simulink model "task3"  (R2017a)
settings: Solver=VariableStepAuto  StartTime=0.0  StopTime=w_base  MaxStep=1e-4*w_base  RelTol=1e-3
values from neighbouring files (symbols this model uses):
  I_base = 1    [parameters.m]
  K = sqrt(3/2)    [parameters.m]    (also in working.m)
  ki = alpha_c*(R+Ra)    (= 11.8344493889)    [parameters.m]
  ki_speed = alpha_speed*alpha_speed*J    (= 24.390868485)    [parameters.m]
  kp = alpha_c*Lsigma    (= 1.69441359229)    [parameters.m]
  kp_speed = alpha_speed*J    (= 34.9219619187)    [parameters.m]
  LM = 1.301    [parameters.m]
  Lsigma = 0.2426    [parameters.m]
  Ra = alpha_c*Lsigma-R    (= 1.58785359229)    [parameters.m]
  Ra_speed = alpha_speed*J-b    (= 34.4219619187)    [parameters.m]
  Tr = LM/RR    (= 21.1510323525)    [parameters.m]
  V_base = 1    [parameters.m]
settings Model: Creator=Oskar  LastModifiedBy=Callum

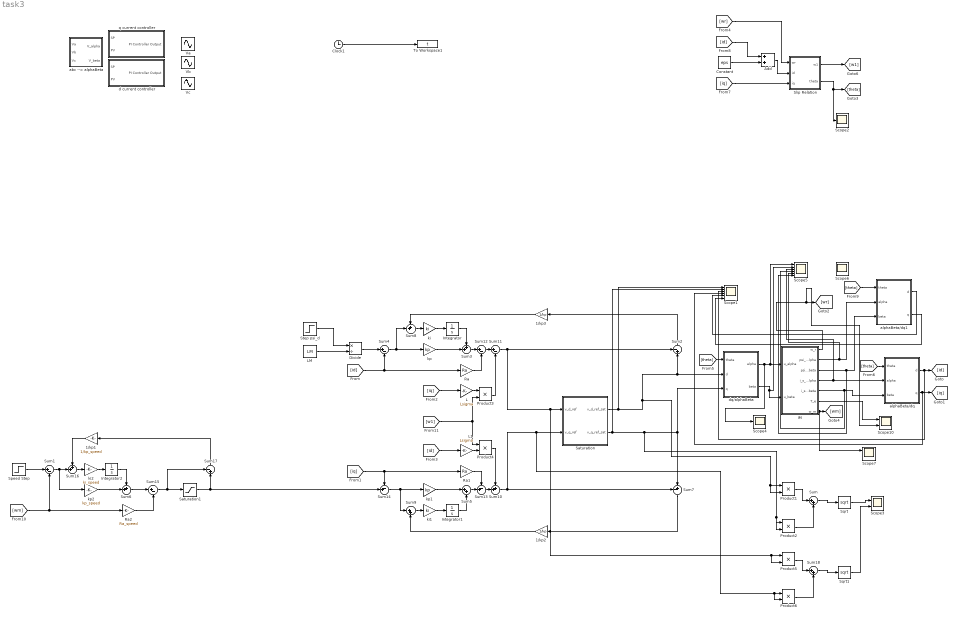
== system task3 ==
  1/kp1 : Gain  Gain=1/kp_speed
  1/kp2 : Gain  Gain=1/kp
  1/kp3 : Gain  Gain=1/kp
  Add : Sum
  Clock1 : Clock
  Constant : Constant  Value=eps
  Divide : Product  Inputs=*/
  IM : Subsystem  mask{RR=0.06151, RS=0.04505, LM=1.301, Ls=0.2426, J=50, p=2, b_w1=0.5, b_w2=0}
      mask prompts: RR "Rr [p.u]"; RS "Rs [p.u]"; LM "Lm [p.u]"; Ls "Ls [p.u]"; J "J [p.u]"
  Integrator : Integrator
  Integrator1 : Integrator
  Integrator2 : Integrator
  L : Gain  Gain=Lsigma
  L1 : Gain  Gain=Lsigma
  LM : Constant  Value=LM
  Product{1..6} (6 alike) : Product
  Ra : Gain  Gain=Ra
  Ra1 : Gain  Gain=Ra
  Ra2 : Gain  Gain=Ra_speed
  Saturation : Subsystem
  Saturation1 : Saturate  UpperLimit=I_base  LowerLimit=-I_base
  Scope1 : Scope  NumInputPorts=6
  Scope10 : Scope  NumInputPorts=2
  Scope2 : Scope
  Scope3 : Scope  NumInputPorts=2
  Scope4 : Scope
  Scope5 : Scope  NumInputPorts=6
  Scope6 : Scope
  Scope7 : Scope  NumInputPorts=2
  Slip Relation : Subsystem
  Speed Step : Step  Time=150  After=0.3  SampleTime=0
  Sqrt : Sqrt  SaturateOnIntegerOverflow=on
  Sqrt1 : Sqrt  SaturateOnIntegerOverflow=on
  Step psi_d : Step  Time=0  Before=1  SampleTime=0
  Sum{,5,9,18} (4 alike) : Sum  Inputs=|++
  Sum{1,4,11..12,15} (5 alike) : Sum  Inputs=|+-
  Sum{3,6,8,10,16} (5 alike) : Sum  Inputs=++|
  Sum{2,7,13..14,17} (5 alike) : Sum  Inputs=-+|
  To Workspace1 : ToWorkspace  VariableName=t
      settings: MaxDataPoints=100000
  Va : Sin  SampleTime=0
  Vb : Sin  Phase=2*pi/3  SampleTime=0
  Vc : Sin  Phase=4*pi/3  SampleTime=0
  abc --> alphaBeta : Subsystem
  alphaBeta/dq : Subsystem
  alphaBeta/dq1 : Subsystem
  d current controller : Subsystem
  dq/alphaBeta : Subsystem
  ki : Gain  Gain=ki
  ki1 : Gain  Gain=ki
  ki2 : Gain  Gain=ki_speed
  kp : Gain  Gain=kp
  kp1 : Gain  Gain=kp
  kp2 : Gain  Gain=kp_speed
  q current controller : Subsystem
  wires:
  Clock1/1 -> To Workspace1/1
  dq/alphaBeta/1(alpha) -> Scope4/1, Scope5/1, IM/1(u_alpha)
  dq/alphaBeta/2(beta) -> Scope5/2, IM/2(u_beta)
  IM/4(i_s_s_alpha) -> Scope5/3, alphaBeta/dq/2(alpha)
  IM/5(i_s_s_beta) -> Scope5/4, alphaBeta/dq/3("beta ")
  alphaBeta/dq/1(d) -> Scope1/3, [id]
  ki/1 -> Integrator/1
  Sum4/1 -> kp/1, Sum8/2
  [id] -> Ra/1, Sum4/2
  Sum14/1 -> kp1/1, Sum9/1
  ki1/1 -> Integrator1/1
  kp1/1 -> Sum5/1
  Integrator1/1 -> Sum5/2
  Sum7/1 -> 1/kp2/1
  Sum2/1 -> 1/kp3/1
  kp/1 -> Sum3/2
  Integrator/1 -> Sum3/1
  Sum8/1 -> ki/1
  1/kp3/1 -> Sum8/1
  Sum9/1 -> ki1/1
  1/kp2/1 -> Sum9/2
  Sum11/1 -> Product5/2, Product5/1, Saturation/1(v_d_ref), Sum2/1
  [iq] -> L/1
  Sum10/1 -> Product6/2, Product6/1, Saturation/2(v_q_ref), Sum7/1
  [id] -> L1/1
  Sum3/1 -> Sum12/1
  Sum12/1 -> Sum11/1
  Ra/1 -> Sum12/2
  Sum5/1 -> Sum13/2
  Sum13/1 -> Sum10/2
  Ra1/1 -> Sum13/1
  [iq] -> Ra1/1, Sum14/1
  [wr] -> Slip Relation/1(wr)
  Slip Relation/2(theta) -> Scope2/1, [theta]
  [theta] -> dq/alphaBeta/1(theta)
  [theta] -> alphaBeta/dq/1(theta)
  [iq] -> Slip Relation/3("iq ")
  L/1 -> Product3/1
  Product3/1 -> Sum11/2
  [w1] -> Product3/2, Product4/1
  L1/1 -> Product4/2
  Product4/1 -> Sum10/1
  Saturation/2(v_q_ref_sat) -> Product2/2, Product2/1, dq/alphaBeta/3("q "), Sum7/2, Scope1/2
  IM/2(psi_r_alpha) -> Scope5/5, alphaBeta/dq1/2(alpha)
  IM/3(psi_r_beta) -> Scope5/6, alphaBeta/dq1/3("beta ")
  [theta] -> alphaBeta/dq1/1(theta)
  Slip Relation/1(w1) -> [w1]
  Add/1 -> Slip Relation/2(id)
  Constant/1 -> Add/2
  [id] -> Add/1
  Speed Step/1 -> Sum1/1
  [wm] -> Sum1/2, Ra2/1
  ki2/1 -> Integrator2/1
  Sum16/1 -> ki2/1
  kp2/1 -> Sum6/2
  Integrator2/1 -> Sum6/1
  Sum1/1 -> kp2/1, Sum16/2
  Sum6/1 -> Sum15/1
  Ra2/1 -> Sum15/2
  1/kp1/1 -> Sum16/1
  Sum15/1 -> Sum17/1, Saturation1/1
  Sum17/1 -> 1/kp1/1
  Sum/1 -> Sqrt/1
  Product1/1 -> Sum/1
  Product2/1 -> Sum/2
  Sqrt/1 -> Scope3/1
  Sum18/1 -> Sqrt1/1
  Product6/1 -> Sum18/2
  Product5/1 -> Sum18/1
  Sqrt1/1 -> Scope3/2
  Divide/1 -> Sum4/1
  Step psi_d/1 -> Divide/1
  LM/1 -> Divide/2
  Saturation/1(v_d_ref_sat) -> Scope1/1, Product1/2, Product1/1, Sum2/2, dq/alphaBeta/2(d)
  alphaBeta/dq/2(q) -> Scope1/4, [iq]
  alphaBeta/dq1/2(q) -> Scope1/6
  alphaBeta/dq1/1(d) -> Scope1/5
  IM/1(w_r) -> Scope10/2, [wr]
  IM/7(w_m) -> Scope7/1, [wm]
  IM/6(T_e) -> Scope10/1
  Saturation1/1 -> Sum14/2, Sum17/2

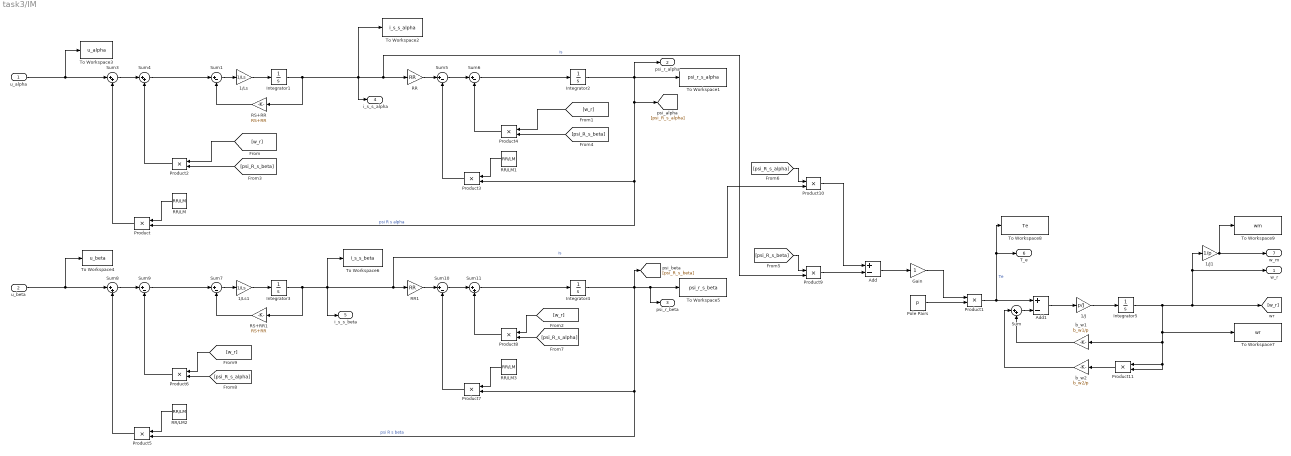
== system task3/IM ==
  u_alpha : Inport
  u_beta : Inport  Port=2
  1/J : Gain  Gain=p/J
  1/J1 : Gain  Gain=1/p
  1/Ls : Gain  Gain=1/Ls
  1/Ls1 : Gain  Gain=1/Ls
  Add : Sum  Inputs=+-
  Add1 : Sum  Inputs=+-
  Gain : Gain
  Integrator{1..5} (5 alike) : Integrator
  Pole Pairs : Constant  Value=p
  Product{,1..11} (12 alike) : Product  SaturateOnIntegerOverflow=on  InputSameDT=on  OutDataTypeStr=Inherit: Same as first input
  RR : Gain  Gain=RR
  RR/LM{,1..3} (4 alike) : Constant  Value=RR/LM
  RR1 : Gain  Gain=RR
  RS+RR : Gain  Gain=RS+RR
  RS+RR1 : Gain  Gain=RS+RR
  Sum{,3..4,8,11} (5 alike) : Sum  Inputs=|++
  Sum{1,5..7,9..10} (6 alike) : Sum  Inputs=|+-
  To Workspace1 : ToWorkspace  VariableName=psi_r_s_alpha
      settings: MaxDataPoints=100000
  To Workspace2 : ToWorkspace  VariableName=i_s_s_alpha
      settings: MaxDataPoints=100000
  To Workspace3 : ToWorkspace  VariableName=u_alpha
      settings: MaxDataPoints=100000
  To Workspace4 : ToWorkspace  VariableName=u_beta
      settings: MaxDataPoints=100000
  To Workspace5 : ToWorkspace  VariableName=psi_r_s_beta
      settings: MaxDataPoints=100000
  To Workspace6 : ToWorkspace  VariableName=i_s_s_beta
      settings: MaxDataPoints=100000
  To Workspace7 : ToWorkspace  VariableName=wr
      settings: MaxDataPoints=100000
  To Workspace8 : ToWorkspace  VariableName=Te
      settings: MaxDataPoints=100000
  To Workspace9 : ToWorkspace  VariableName=wm
      settings: MaxDataPoints=100000
  b_w1 : Gain  Gain=b_w1/p
  b_w2 : Gain  Gain=b_w2/p
  w_r : Outport
  psi_r_alpha : Outport  Port=2
  psi_r_beta : Outport  Port=3
  i_s_s_alpha : Outport  Port=4
  i_s_s_beta : Outport  Port=5
  T_e : Outport  Port=6
  w_m : Outport  Port=7
  wires:
  RR/LM1/1 -> Product3/1
  Product3/1 -> Sum5/2
  [psi_R_s_alpha] -> Product8/2
  1/Ls/1 -> Integrator1/1
  1/J/1 -> Integrator5/1
  Pole Pairs/1 -> Product1/2
  Add1/1 -> 1/J/1
  Sum1/1 -> 1/Ls/1
  Sum3/1 -> Sum4/1
  Sum4/1 -> Sum1/1
  Integrator2/1 -> psi_r_alpha/1, [psi_R_s_alpha], Product/2, Product3/2, To Workspace1/1  "psi R s alpha"
  RR/LM/1 -> Product/1
  Product10/1 -> Add/1
  Product9/1 -> Add/2
  Sum5/1 -> Sum6/1
  [psi_R_s_beta] -> Product2/2
  [w_r] -> Product2/1
  [w_r] -> Product6/1
  Product/1 -> Sum3/2
  Product1/1 -> To Workspace8/1, T_e/1, Add1/1  "Te"
  [w_r] -> Product8/1
  Sum6/1 -> Integrator2/1
  Add/1 -> Gain/1
  Product5/1 -> Sum8/2
  Sum11/1 -> Integrator4/1
  Integrator3/1 -> i_s_s_beta/1, Product10/2, RR1/1, To Workspace6/1, RS+RR1/1  "is"
  RR/LM3/1 -> Product7/1
  Sum9/1 -> Sum7/1
  RS+RR1/1 -> Sum7/2
  1/Ls1/1 -> Integrator3/1
  Sum8/1 -> Sum9/1
  Integrator4/1 -> [psi_R_s_beta], Product5/2, Product7/2, psi_r_beta/1, To Workspace5/1  "psi R s beta"
  RR1/1 -> Sum10/1
  Product8/1 -> Sum11/2
  u_beta/1 -> To Workspace4/1, Sum8/1
  Product6/1 -> Sum9/2
  Product7/1 -> Sum10/2
  Sum10/1 -> Sum11/1
  RR/LM2/1 -> Product5/1
  Sum7/1 -> 1/Ls1/1
  [psi_R_s_beta] -> Product9/1
  Integrator1/1 -> i_s_s_alpha/1, Product9/2, RR/1, To Workspace2/1, RS+RR/1  "is"
  Product4/1 -> Sum6/2
  u_alpha/1 -> Sum3/1, To Workspace3/1
  Gain/1 -> Product1/1
  [w_r] -> Product4/1
  [psi_R_s_alpha] -> Product10/1
  [psi_R_s_alpha] -> Product6/2
  [psi_R_s_beta] -> Product4/2
  RR/1 -> Sum5/1
  RS+RR/1 -> Sum1/2
  Product2/1 -> Sum4/2
  Sum/1 -> Add1/2
  b_w1/1 -> Sum/2
  b_w2/1 -> Sum/1
  Product11/1 -> b_w2/1
  Integrator5/1 -> 1/J1/1, w_r/1, [w_r], Product11/2, Product11/1, b_w1/1, To Workspace7/1
  1/J1/1 -> To Workspace9/1, w_m/1

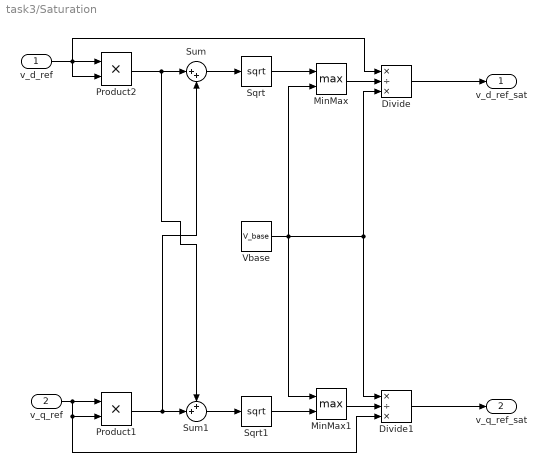
== system task3/Saturation ==
  v_d_ref : Inport
  v_q_ref : Inport  Port=2
  Divide : Product  Inputs=*/*
  Divide1 : Product  Inputs=*/*
  MinMax : MinMax  Function=max  Inputs=2
  MinMax1 : MinMax  Function=max  Inputs=2
  Product1 : Product
  Product2 : Product
  Sqrt : Sqrt  SaturateOnIntegerOverflow=on
  Sqrt1 : Sqrt  SaturateOnIntegerOverflow=on
  Sum : Sum  Inputs=|++
  Sum1 : Sum  Inputs=++|
  Vbase : Constant  Value=V_base
  v_d_ref_sat : Outport
  v_q_ref_sat : Outport  Port=2
  wires:
  Sum1/1 -> Sqrt1/1
  MinMax1/1 -> Divide1/2
  Sum/1 -> Sqrt/1
  Product2/1 -> Sum/1, Sum1/1
  MinMax/1 -> Divide/2
  Sqrt1/1 -> MinMax1/2
  Vbase/1 -> MinMax/2, Divide/3, Divide1/1, MinMax1/1
  Divide/1 -> v_d_ref_sat/1
  Divide1/1 -> v_q_ref_sat/1
  Product1/1 -> Sum/2, Sum1/2
  Sqrt/1 -> MinMax/1
  v_d_ref/1 -> Divide/1, Product2/2, Product2/1
  v_q_ref/1 -> Divide1/3, Product1/2, Product1/1

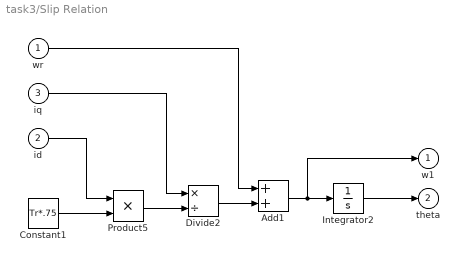
== system task3/Slip Relation ==
  wr : Inport
  id : Inport  Port=2
  "iq " : Inport  Port=3
  Add1 : Sum
  Constant1 : Constant  Value=Tr*.75
  Divide2 : Product  Inputs=*/
  Integrator2 : Integrator
  Product5 : Product
  w1 : Outport
  theta : Outport  Port=2
  wires:
  Constant1/1 -> Product5/2
  Divide2/1 -> Add1/2
  id/1 -> Product5/1
  Add1/1 -> w1/1, Integrator2/1
  Integrator2/1 -> theta/1
  "iq "/1 -> Divide2/1
  wr/1 -> Add1/1
  Product5/1 -> Divide2/2

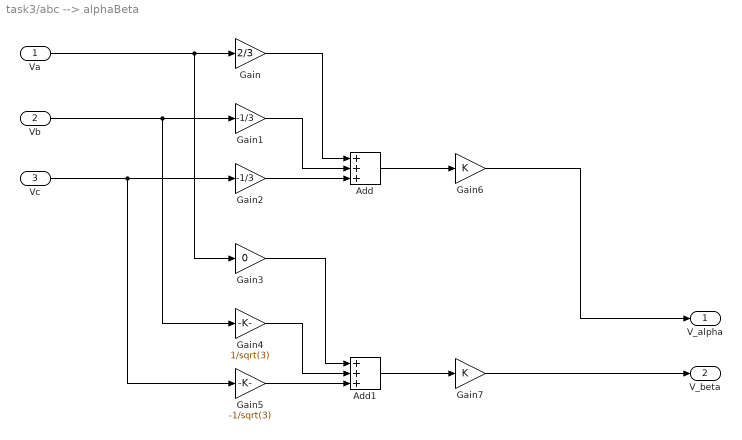
== system task3/abc --> alphaBeta ==
  Va : Inport
  Vb : Inport  Port=2
  Vc : Inport  Port=3
  Add : Sum  Inputs=+++
  Add1 : Sum  Inputs=+++
  Gain : Gain  Gain=2/3
  Gain1 : Gain  Gain=-1/3
  Gain2 : Gain  Gain=-1/3
  Gain3 : Gain  Gain=0
  Gain4 : Gain  Gain=1/sqrt(3)
  Gain5 : Gain  Gain=-1/sqrt(3)
  Gain6 : Gain  Gain=K
  Gain7 : Gain  Gain=K
  V_alpha : Outport
  V_beta : Outport  Port=2
  wires:
  Add/1 -> Gain6/1
  Va/1 -> Gain3/1, Gain/1
  Vc/1 -> Gain5/1, Gain2/1
  Vb/1 -> Gain4/1, Gain1/1
  Gain3/1 -> Add1/1
  Gain6/1 -> V_alpha/1
  Gain7/1 -> V_beta/1
  Add1/1 -> Gain7/1
  Gain1/1 -> Add/2
  Gain/1 -> Add/1
  Gain5/1 -> Add1/3
  Gain2/1 -> Add/3
  Gain4/1 -> Add1/2

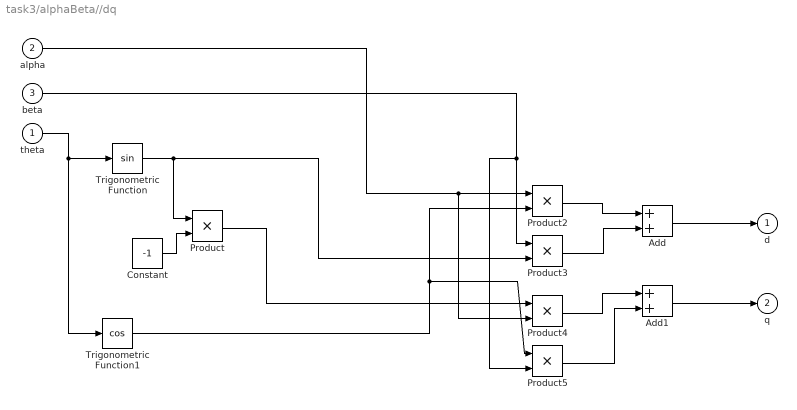
== system task3/alphaBeta//dq ==
  theta : Inport
  alpha : Inport  Port=2
  "beta " : Inport  Port=3
  Add : Sum
  Add1 : Sum
  Constant : Constant  Value=-1
  Product{,2..5} (5 alike) : Product
  Trigonometric Function : Trigonometry
  Trigonometric Function1 : Trigonometry  Operator=cos
  d : Outport
  q : Outport  Port=2
  wires:
  theta/1 -> Trigonometric Function1/1, Trigonometric Function/1
  Product4/1 -> Add1/1
  Product5/1 -> Add1/2
  Trigonometric Function1/1 -> Product2/2, Product5/1
  Product/1 -> Product4/1
  Trigonometric Function/1 -> Product/1, Product3/2
  Add1/1 -> q/1
  alpha/1 -> Product2/1, Product4/2
  "beta "/1 -> Product5/2, Product3/1
  Add/1 -> d/1
  Constant/1 -> Product/2
  Product2/1 -> Add/1
  Product3/1 -> Add/2

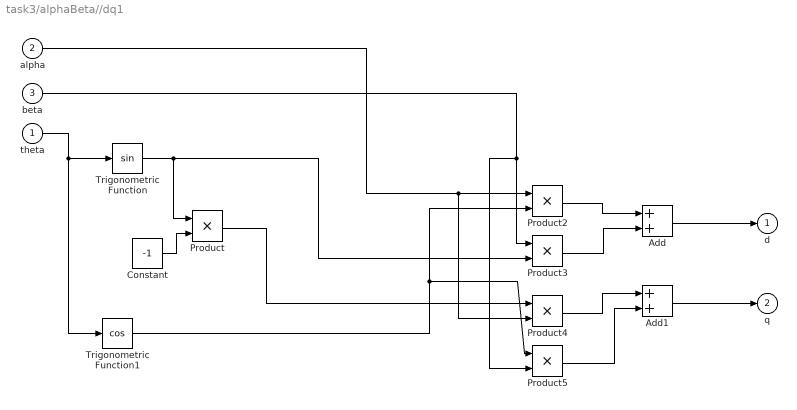
== system task3/alphaBeta//dq1 ==
  theta : Inport
  alpha : Inport  Port=2
  "beta " : Inport  Port=3
  Add : Sum
  Add1 : Sum
  Constant : Constant  Value=-1
  Product{,2..5} (5 alike) : Product
  Trigonometric Function : Trigonometry
  Trigonometric Function1 : Trigonometry  Operator=cos
  d : Outport
  q : Outport  Port=2
  wires:
  theta/1 -> Trigonometric Function1/1, Trigonometric Function/1
  Product4/1 -> Add1/1
  Product5/1 -> Add1/2
  Trigonometric Function1/1 -> Product2/2, Product5/1
  Product/1 -> Product4/1
  Trigonometric Function/1 -> Product/1, Product3/2
  Add1/1 -> q/1
  alpha/1 -> Product2/1, Product4/2
  "beta "/1 -> Product5/2, Product3/1
  Add/1 -> d/1
  Constant/1 -> Product/2
  Product2/1 -> Add/1
  Product3/1 -> Add/2

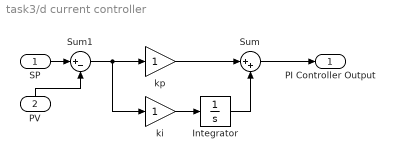
== system task3/d current controller ==
  SP : Inport
  PV : Inport  Port=2
  Integrator : Integrator
  Sum : Sum  Inputs=|++
  Sum1 : Sum  Inputs=|+-
  ki : Gain
  kp : Gain
  PI Controller Output : Outport
  wires:
  ki/1 -> Integrator/1
  kp/1 -> Sum/1
  Integrator/1 -> Sum/2
  Sum/1 -> PI Controller Output/1
  Sum1/1 -> ki/1, kp/1
  PV/1 -> Sum1/2
  SP/1 -> Sum1/1

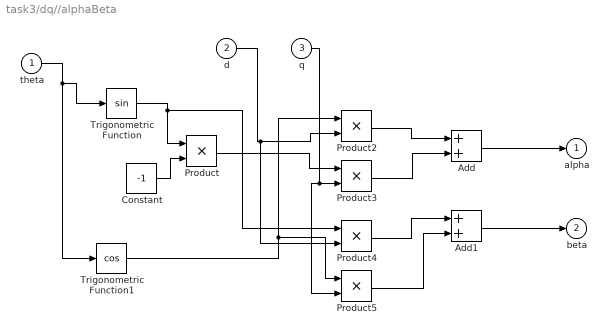
== system task3/dq//alphaBeta ==
  theta : Inport
  d : Inport  Port=2
  "q " : Inport  Port=3
  Add : Sum
  Add1 : Sum
  Constant : Constant  Value=-1
  Product{,2..5} (5 alike) : Product
  Trigonometric Function : Trigonometry
  Trigonometric Function1 : Trigonometry  Operator=cos
  alpha : Outport
  beta : Outport  Port=2
  wires:
  theta/1 -> Trigonometric Function1/1, Trigonometric Function/1
  Product4/1 -> Add1/1
  Product5/1 -> Add1/2
  Trigonometric Function/1 -> Product4/1, Product/1
  Add1/1 -> beta/1
  Add/1 -> alpha/1
  Constant/1 -> Product/2
  Product2/1 -> Add/1
  Product3/1 -> Add/2
  Trigonometric Function1/1 -> Product5/1, Product2/1
  Product/1 -> Product3/1
  d/1 -> Product4/2, Product2/2
  "q "/1 -> Product3/2, Product5/2

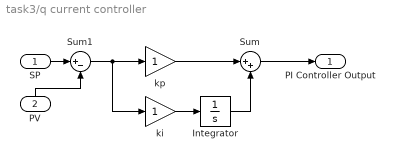
== system task3/q current controller ==
  SP : Inport
  PV : Inport  Port=2
  Integrator : Integrator
  Sum : Sum  Inputs=|++
  Sum1 : Sum  Inputs=|+-
  ki : Gain
  kp : Gain
  PI Controller Output : Outport
  wires:
  ki/1 -> Integrator/1
  kp/1 -> Sum/1
  Integrator/1 -> Sum/2
  Sum/1 -> PI Controller Output/1
  Sum1/1 -> ki/1, kp/1
  PV/1 -> Sum1/2
  SP/1 -> Sum1/1
